simulink model "Mealy_Vending_Machine"  (R2020b)
settings: Solver=VariableStepAuto  StartTime=0.0  StopTime=10.0  RelTol=1e-3
settings Model: Creator=HP  LastModifiedBy=HP

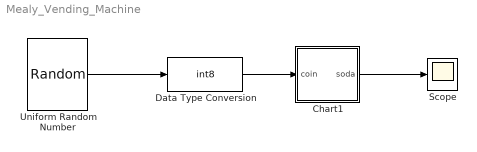
== system Mealy_Vending_Machine ==
  Chart1 : Stateflow chart  TreatAsAtomicUnit=on
  Data Type Conversion : DataTypeConversion  OutDataTypeStr=int8  RndMeth=Nearest  SaturateOnIntegerOverflow=on
  Scope : Scope
  Uniform Random Number : UniformRandomNumber  Minimum=0  Maximum=2  Seed=337  SampleTime=10
  wires:
  Chart1/1(soda) -> Scope/1
  Data Type Conversion/1 -> Chart1/1(coin)
  Uniform Random Number/1 -> Data Type Conversion/1

== stateflow chart Mealy_Vending_Machine/Chart1 ==
  state got_nickel
  state got_0
  state got_dime
  (default) -> got_0
  got_0 -> got_nickel [order 1] : [coint==1]{soda=0}
  got_nickel -> got_0 [order 2] : [coin==2]{soda=1}
  got_dime -> got_0 [order 1] : [coin==1]{soda=1}
  got_0 -> got_dime [order 2] : [coin==1]{soda=0}
  got_nickel -> got_dime [order 1] : [coin==1]{soda=0}
  got_dime -> got_nickel [order 2] : [coin==2]{soda=1}
  data: coin input; coint local; soda output
